simulink model "Braking_dynamic"  (R2024b)
settings: Solver=VariableStepAuto  StartTime=0.0  StopTime=10.0  RelTol=1e-3
values from neighbouring files (symbols this model uses):
  brake_repartition = 0.6    [braking_dyn.m]
  vehicle = struct    [model2_dim.m]
libraries: simulink x1
settings Model: Creator=francescovalentia  LastModifiedBy=francescovalentia

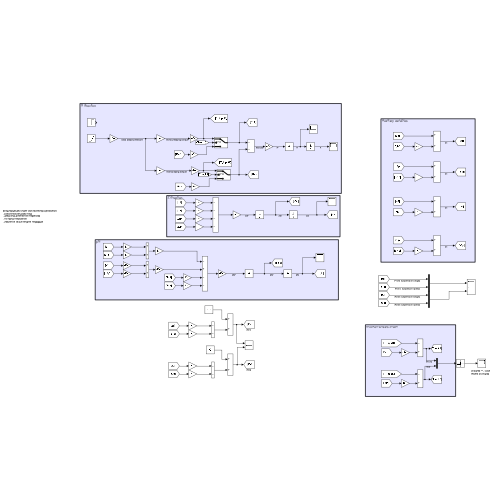
[thumbnail: Simulink's stored preview of the top-level diagram]
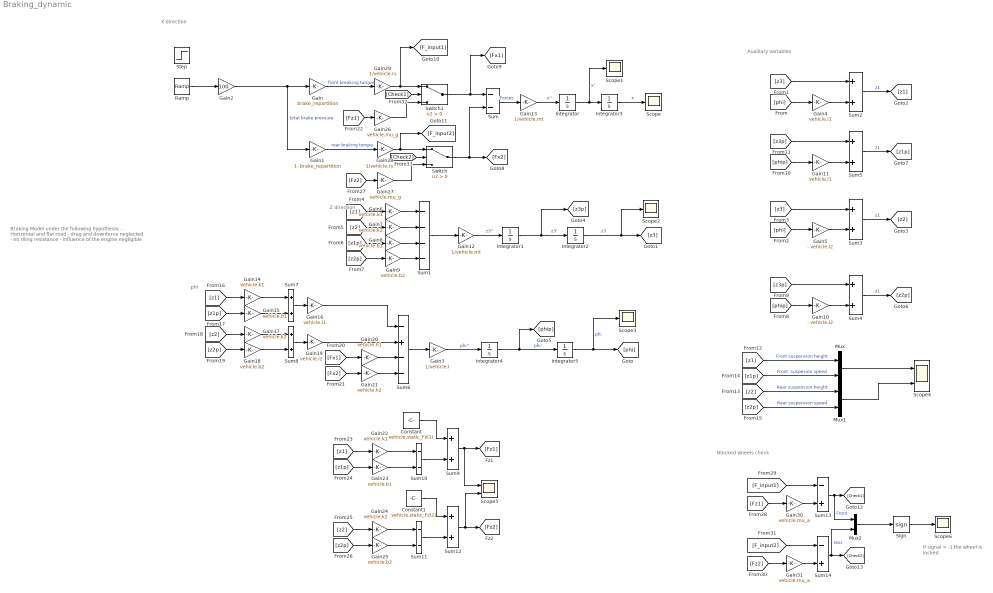
== system Braking_dynamic ==
  note: If signal = -1 the wheel is locked
  note: Z direction
  note: phi
  note: X direction
  note: Auxiliary variables
  note: Blocked wheels check
  note: Braking Model under the following hypothesis:
      | - Horizontal and flat road
      | - drag and downforce neglected
      | - no rlling resistance
      | - influence of the engine negligible
  Constant : Constant  Value=vehicle.static_Fz(1)  VectorParams1D=off
  Constant1 : Constant  Value=vehicle.static_Fz(2)  VectorParams1D=off
  Gain : Gain  Gain=brake_repartition
  Gain1 : Gain  Gain=1- brake_repartition
  Gain10 : Gain  Gain=- vehicle.l2
  Gain11 : Gain  Gain=vehicle.l1
  Gain12 : Gain  Gain=1/vehicle.mt
  Gain13 : Gain  Gain=1/vehicle.mt
  Gain14 : Gain  Gain=vehicle.k1
  Gain15 : Gain  Gain=vehicle.b1
  Gain16 : Gain  Gain=vehicle.l1
  Gain17 : Gain  Gain=vehicle.k2
  Gain18 : Gain  Gain=vehicle.b2
  Gain19 : Gain  Gain=vehicle.l2
  Gain2 : Gain  Gain=100
  Gain20 : Gain  Gain=vehicle.h1
  Gain21 : Gain  Gain=vehicle.h2
  Gain22 : Gain  Gain=vehicle.k1
  Gain23 : Gain  Gain=vehicle.b1
  Gain24 : Gain  Gain=vehicle.k2
  Gain25 : Gain  Gain=vehicle.b2
  Gain26 : Gain  Gain=vehicle.mu_g
  Gain27 : Gain  Gain=vehicle.mu_g
  Gain28 : Gain  Gain=1/vehicle.rs
  Gain29 : Gain  Gain=1/vehicle.rs
  Gain3 : Gain  Gain=1/vehicle.I
  Gain30 : Gain  Gain=vehicle.mu_a
  Gain31 : Gain  Gain=vehicle.mu_a
  Gain4 : Gain  Gain=vehicle.l1
  Gain5 : Gain  Gain=- vehicle.l2
  Gain6 : Gain  Gain=vehicle.k1
  Gain7 : Gain  Gain=vehicle.k2
  Gain8 : Gain  Gain=vehicle.b1
  Gain9 : Gain  Gain=vehicle.b2
  Integrator : Integrator  InitialCondition=100
  Integrator{1..5} (5 alike) : Integrator
  Mux : Mux  Inputs=2
  Mux1 : Mux  Inputs=2
  Mux2 : Mux  Inputs=2
  Ramp : simulink/Sources/Ramp  slope=0.4  start=0  InitialOutput=0
  Scope{,1..3,6} (5 alike) : Scope
  Scope4 : Scope  NumInputPorts=2
  Scope5 : Scope  NumInputPorts=2
  Sign : Signum
  Step : Step  SampleTime=0
  Sum : Sum  Inputs=--
  Sum1 : Sum  Inputs=----
  Sum10 : Sum  Inputs=--
  Sum11 : Sum  Inputs=--
  Sum{2..5,7..9,12} (8 alike) : Sum
  Sum13 : Sum  Inputs=-+
  Sum14 : Sum  Inputs=-+
  Sum6 : Sum  Inputs=-+--
  Switch : Switch  Criteria=u2 > Threshold  SaturateOnIntegerOverflow=off  InputSameDT=off
  Switch1 : Switch  Criteria=u2 > Threshold  SaturateOnIntegerOverflow=off  InputSameDT=off
  wires:
  Gain1/1 -> Gain28/1  "rear braking torque"
  Gain2/1 -> Gain/1, Gain1/1  "total brake pressure"
  Integrator1/1 -> [z3p], Integrator2/1  "z3'"
  Integrator2/1 -> Scope2/1, [z3]  "z3"
  Integrator/1 -> Scope1/1, Integrator3/1  "x'"
  Integrator3/1 -> Scope/1  "x"
  Sum2/1 -> [z1]  "z1"
  Integrator4/1 -> [phip], Integrator5/1  "phi'"
  Integrator5/1 -> Scope3/1, [phi]  "phi"
  Gain3/1 -> Integrator4/1  "phi''"
  [z3] -> Sum2/1
  [phi] -> Gain4/1
  Gain4/1 -> Sum2/2
  [z3] -> Sum3/1
  Gain5/1 -> Sum3/2
  Sum3/1 -> [z2]  "z1"
  [phi] -> Gain5/1
  [z1] -> Gain6/1
  Gain6/1 -> Sum1/1
  [z2] -> Gain7/1
  Gain7/1 -> Sum1/2
  [z1p] -> Gain8/1
  Gain8/1 -> Sum1/3
  [z2p] -> Gain9/1
  Gain9/1 -> Sum1/4
  [z3p] -> Sum4/1
  Sum4/1 -> [z2p]  "z1"
  [phip] -> Gain10/1
  Gain10/1 -> Sum4/2
  [z3p] -> Sum5/1
  Sum5/1 -> [z1p]  "z1"
  [phip] -> Gain11/1
  Gain11/1 -> Sum5/2
  Sum1/1 -> Gain12/1
  Gain12/1 -> Integrator1/1  "z3''"
  Gain/1 -> Gain29/1  "front breaking torque"
  Sum/1 -> Gain13/1  "Forces"
  Gain13/1 -> Integrator/1  "x''"
  Sum6/1 -> Gain3/1
  [z1] -> Gain14/1
  Gain14/1 -> Sum7/1
  [z1p] -> Gain15/1
  Gain15/1 -> Sum7/2
  Sum7/1 -> Gain16/1
  Gain18/1 -> Sum8/2
  Gain17/1 -> Sum8/1
  Sum8/1 -> Gain19/1
  [z2p] -> Gain18/1
  [z2] -> Gain17/1
  Gain19/1 -> Sum6/2
  Gain16/1 -> Sum6/1
  Switch/1 -> [Fx2], Sum/2
  Switch1/1 -> [Fx1], Sum/1
  [Fx1] -> Gain20/1
  Gain20/1 -> Sum6/3
  Gain21/1 -> Sum6/4
  [Fx2] -> Gain21/1
  Constant/1 -> Sum9/1
  Sum9/1 -> Scope5/1, [Fz1]
  Gain23/1 -> Sum10/2
  Gain22/1 -> Sum10/1
  Sum10/1 -> Sum9/2
  [z1p] -> Gain23/1
  [z1] -> Gain22/1
  [z2p] -> Gain25/1
  Gain25/1 -> Sum11/2
  Gain24/1 -> Sum11/1
  [z2] -> Gain24/1
  Constant1/1 -> Sum12/1
  Sum11/1 -> Sum12/2
  Sum12/1 -> Scope5/2, [Fz2]
  [Fz1] -> Gain26/1
  Gain26/1 -> Switch1/3
  [Fz2] -> Gain27/1
  Gain27/1 -> Switch/3
  Gain28/1 -> [F_input2], Switch/1
  Gain29/1 -> [F_input1], Switch1/1
  [Fz1] -> Gain30/1
  Gain30/1 -> Sum13/2
  [F_input1] -> Sum13/1
  [Fz2] -> Gain31/1
  [F_input2] -> Sum14/1
  Gain31/1 -> Sum14/2
  Sum13/1 -> Mux2/1, [Check1]  "Front"
  Sum14/1 -> Mux2/2, [Check2]  "rear"
  [Check1] -> Switch1/2
  [Check2] -> Switch/2
  Ramp/1 -> Gain2/1
  [z1] -> Mux/1  "Front suspension height"
  Mux/1 -> Scope4/1
  Mux1/1 -> Scope4/2
  [z2p] -> Mux1/2  "Rear suspension speed"
  [z1p] -> Mux/2  "Front  suspesion speed"
  [z2] -> Mux1/1  "Rear suspension height"
  Sign/1 -> Scope6/1
  Mux2/1 -> Sign/1
